simulink model "SimulinkP8_1"  (R2018b)
settings: Solver=VariableStepAuto  StartTime=0.0  StopTime=30  RelTol=1e-3
values from neighbouring files (symbols this model uses):
  C = [ 1 0 ]    [Problema8_1.m]
  C2 = [0 1]    [Problema8_1.m]
  Ca = [ 1 0; 0 1 ]    [Problema8_1.m]
  Da = [ 0; 0 ]    [Problema8_1.m]
  gama = [ 2; 1 ]    [Problema8_1.m]
  h = Wnh/Wn    [Problema8_1.m]
  L = [0 1] * inv(Wc)*(phi^2 + p1*phi + p2*eye(2))    [Problema8_1.m]
  Lc = ganho_dc/( C*inv( eye(2) - phi_cl )*gama )    [Problema8_1.m]
  phi = [1 Phi12; 0 0.4]    [Problema8_1.m]
settings Model: Creator=root  LastModifiedBy=root

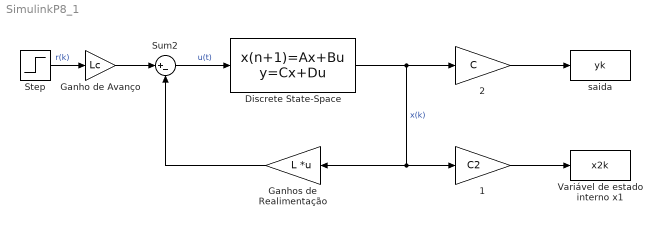
== system SimulinkP8_1 ==
  " saida" : ToWorkspace  VariableName=yk  SaveFormat=Structure With Time  SampleTime=-1
  1 : Gain  Gain=C2
  2 : Gain  Gain=C
  Discrete State-Space : DiscreteStateSpace  A=phi  B=gama  C=Ca  D=Da  SampleTime=h
  Ganho de Avanço : Gain  Gain=Lc
  Ganhos de Realimentação : Gain  Gain=L  Multiplication=Matrix(K*u)
  Step : Step  Time=0  SampleTime=0
  Sum2 : Sum  Inputs=|+-
  Variável de estado interno x1 : ToWorkspace  VariableName=x2k  SaveFormat=Structure With Time  SampleTime=-1
  wires:
  Ganhos de Realimentação/1 -> Sum2/2
  Ganho de Avanço/1 -> Sum2/1
  Step/1 -> Ganho de Avanço/1  "r(k)"
  Sum2/1 -> Discrete State-Space/1  "u(t)"
  Discrete State-Space/1 -> Ganhos de Realimentação/1, 1/1, 2/1  "x(k)"
  1/1 -> Variável de estado interno x1/1
  2/1 -> " saida"/1
